simulink model "prob_5"  (R2019b)
settings: Solver=VariableStepAuto  StartTime=0.0  StopTime=10.0  RelTol=1e-3
settings Model: Creator=kcalp  LastModifiedBy=kcalp

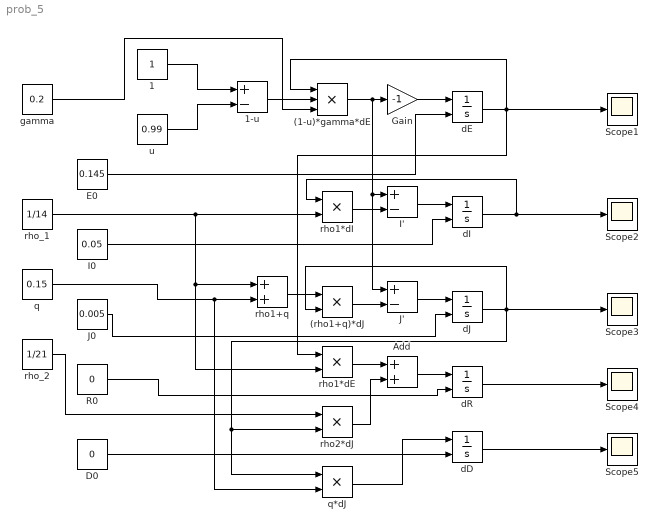
== system prob_5 ==
  (1-u)*gamma*dE : Product  Inputs=3
  "(rho1+q)*dJ " : Product
  "1 " : Constant
  "1-u " : Sum  Inputs=+-
  Add : Sum
  "D0 " : Constant  Value=0
  "E0 " : Constant  Value=0.145
  Gain : Gain  Gain=-1
  I' : Sum  Inputs=+-
  "I0 " : Constant  Value=0.05
  J' : Sum  Inputs=+-
  "J0 " : Constant  Value=0.005
  "R0 " : Constant  Value=0
  Scope{1..5} (5 alike) : Scope
  dD : Integrator  InitialConditionSource=external
  dE : Integrator  InitialConditionSource=external
  dI : Integrator  InitialConditionSource=external
  dJ : Integrator  InitialConditionSource=external
  dR : Integrator  InitialConditionSource=external
  "gamma " : Constant  Value=0.2
  q : Constant  Value=0.15
  q*dJ : Product
  rho1*dE : Product
  rho1*dI : Product
  "rho1+q " : Sum
  rho2*dJ : Product
  rho_1 : Constant  Value=1/14
  "rho_2 " : Constant  Value=1/21
  "u " : Constant  Value=0.99
  wires:
  dE/1 -> rho1*dE/1, Scope1/1, (1-u)*gamma*dE/1
  "E0 "/1 -> dE/2
  "gamma "/1 -> (1-u)*gamma*dE/3
  "1 "/1 -> "1-u "/1
  "u "/1 -> "1-u "/2
  (1-u)*gamma*dE/1 -> J'/1, I'/1, Gain/1
  Gain/1 -> dE/1
  "1-u "/1 -> (1-u)*gamma*dE/2
  rho1*dI/1 -> I'/2
  dI/1 -> Scope2/1, rho1*dI/1
  rho_1/1 -> rho1*dI/2, "rho1+q "/1, rho1*dE/2
  I'/1 -> dI/1
  "I0 "/1 -> dI/2
  q/1 -> q*dJ/2, "rho1+q "/2
  "rho1+q "/1 -> "(rho1+q)*dJ "/1
  dJ/1 -> "(rho1+q)*dJ "/2, rho2*dJ/2, q*dJ/1, Scope3/1
  "(rho1+q)*dJ "/1 -> J'/2
  J'/1 -> dJ/1
  "J0 "/1 -> dJ/2
  "rho_2 "/1 -> rho2*dJ/1
  rho2*dJ/1 -> Add/2
  rho1*dE/1 -> Add/1
  Add/1 -> dR/1
  "R0 "/1 -> dR/2
  dR/1 -> Scope4/1
  q*dJ/1 -> dD/1
  "D0 "/1 -> dD/2
  dD/1 -> Scope5/1
